simulink model "wlan_phy_tx_pmd"  (Simulink 7.8)
settings: Solver=VariableStepDiscrete  SolverMode=SingleTasking  StartTime=0.0  StopTime=inf  RelTol=1e-3
PostLoadFcn:
  | wlan_phy_tx_init
InitFcn:
  | wlan_phy_tx_init
StartFcn:
  | wlan_phy_tx_init
undefined symbols (not defined in the file): gcbh, ht_preamble_rom, MAX_CP_LEN, MAX_DATA_BITS_PER_SYM_PERIOD, MAX_NCBPS, MAX_NUM_BYTES, MAX_NUM_SC, MAX_NUM_SYMS, mcs_rom_11ag, mcs_rom_11n, Mod_Constellation_16QAM, Mod_Constellation_64QAM, Mod_Constellation_BPSK, Mod_Constellation_QPSK, Preamble_IQ, Preamble_IQ_scaled, tx_sim, wlan_tx_interleave_rom, xlBlockLoadCallback, xlGetNormalizedPeriod
libraries: xbsIndex_r4 x1358, xbsEDKLib_r4 x1
(part 7 of 10)

== system wlan_phy_tx_pmd/PSDU Syms Gen/Pkt Data/Packet Sections ==
  note: 11ag Bytes (L = SIGNAL.LENGTH):
      | 0:2        : SIGNAL       No FCS, Unscrambled
      | 3:4        : SERVICE      No FCS, Scrambled
      | 4:(L-5)    : MAC payload  FCS, Scrambled
      | (L-4):(L-1): FCS          Scrambled
      |            : PAD (zeros)  Unscrambled
      |            : TAIL (zeros) Scrambled
  note: 11n Bytes (L = HT-SIG.LENGTH):
      | 0:2        : SIGNAL       No FCS, Unscrambled
      | 3:8        : HT-SIG       No FCS, Unscrambled
      | 9:10       : SERVICE      No FCS, Scrambled
      | 10:(L-5)   : MAC payload  FCS, Scrambled
      | (L-4):(L-1): FCS          Scrambled
      |            : PAD (zeros)  Unscrambled
      |            : TAIL (zeros) Scrambled
  note: 6 bits past L are unscrambled zero (TAIL).
      | All further bits to fill symbol are scrambled
      | zeros (PAD).
  note: len(SIGNAL)
  note: len(L-SIG + HT-SIG)
  note: len(SERVICE)
  note: len(FCS)
  note: len(TAIL)
  Bit sel : Inport
  Byte Ind : Inport  Port=2
  AddSub1 : xbsIndex_r4/AddSub  mode=Addition  use_carryin=off  use_carryout=off  en=off  latency=1  precision=Full  arith_type=Unsigned  n_bits=ceil(log2(MAX_NUM_BYTES))  bin_pt=0  quantization=Truncate  overflow=Saturate  dbl_ovrd=off  use_behavioral_HDL=off  hw_selection=Fabric  pipelined=off  block_type=addsub
  AddSub2 : xbsIndex_r4/AddSub  mode=Subtraction  use_carryin=off  use_carryout=off  en=off  latency=1  precision=Full  arith_type=Unsigned  n_bits=ceil(log2(MAX_NUM_BYTES))  bin_pt=0  quantization=Truncate  overflow=Saturate  dbl_ovrd=off  use_behavioral_HDL=off  hw_selection=Fabric  pipelined=off  block_type=addsub
  AddSub3 : xbsIndex_r4/AddSub  mode=Addition  use_carryin=off  use_carryout=off  en=off  latency=1  precision=Full  arith_type=Unsigned  n_bits=ceil(log2(MAX_NUM_BYTES))  bin_pt=0  quantization=Truncate  overflow=Saturate  dbl_ovrd=off  use_behavioral_HDL=off  hw_selection=Fabric  pipelined=off  block_type=addsub
  Constant1 : xbsIndex_r4/Constant  const=3  gui_display_data_type=Fixed-point  arith_type=Unsigned  n_bits=3  bin_pt=0  preci_type=Single  exp_width=8  frac_width=24  explicit_period=off  period=1  equ=P=C  opselect=C  inp2=PCIN>>17  opr=+  inp1=P  carry=CIN  dbl_ovrd=off  block_type=constant
  Constant2 : xbsIndex_r4/Constant  const=9  gui_display_data_type=Fixed-point  arith_type=Unsigned  n_bits=4  bin_pt=0  preci_type=Single  exp_width=8  frac_width=24  explicit_period=off  period=1  equ=P=C  opselect=C  inp2=PCIN>>17  opr=+  inp1=P  carry=CIN  dbl_ovrd=off  block_type=constant
  Constant3 : xbsIndex_r4/Constant  const=4  gui_display_data_type=Fixed-point  arith_type=Unsigned  n_bits=3  bin_pt=0  preci_type=Single  exp_width=8  frac_width=24  explicit_period=off  period=1  equ=P=C  opselect=C  inp2=PCIN>>17  opr=+  inp1=P  carry=CIN  dbl_ovrd=off  block_type=constant
  Constant4 : xbsIndex_r4/Constant  const=6  gui_display_data_type=Fixed-point  arith_type=Unsigned  n_bits=3  bin_pt=0  preci_type=Single  exp_width=8  frac_width=24  explicit_period=off  period=1  equ=P=C  opselect=C  inp2=PCIN>>17  opr=+  inp1=P  carry=CIN  dbl_ovrd=off  block_type=constant
  Constant5 : xbsIndex_r4/Constant  const=2  gui_display_data_type=Fixed-point  arith_type=Unsigned  n_bits=3  bin_pt=0  preci_type=Single  exp_width=8  frac_width=24  explicit_period=off  period=1  equ=P=C  opselect=C  inp2=PCIN>>17  opr=+  inp1=P  carry=CIN  dbl_ovrd=off  block_type=constant
  Constant6 : xbsIndex_r4/Constant  const=9  gui_display_data_type=Fixed-point  arith_type=Unsigned  n_bits=4  bin_pt=0  preci_type=Single  exp_width=8  frac_width=24  explicit_period=off  period=1  equ=P=C  opselect=C  inp2=PCIN>>17  opr=+  inp1=P  carry=CIN  dbl_ovrd=off  block_type=constant
  Constant7 : xbsIndex_r4/Constant  const=3  gui_display_data_type=Fixed-point  arith_type=Unsigned  n_bits=4  bin_pt=0  preci_type=Single  exp_width=8  frac_width=24  explicit_period=off  period=1  equ=P=C  opselect=C  inp2=PCIN>>17  opr=+  inp1=P  carry=CIN  dbl_ovrd=off  block_type=constant
  DATA Sections : Scope  NumInputPorts=7
      settings: YMin=-5~-5~-5~-5~-5~-5~-5  YMax=5~5~5~5~5~5~5
  Display : Display
  Gateway Out{1..7} (7 alike) : xbsIndex_r4/Gateway Out  inherit_from_input=off  hdl_port=off  timing_constraint=None  locs_specified=off  LOCs={}  UseAsDAC=off  DACChannel='1'  block_type=gatewayout
  Inverter : xbsIndex_r4/Inverter  en=off  latency=0  dbl_ovrd=off  block_type=inv
  Inverter1 : xbsIndex_r4/Inverter  en=off  latency=0  dbl_ovrd=off  block_type=inv
  Logical1 : xbsIndex_r4/Logical  logical_function=OR  inputs=2  en=off  latency=0  precision=Full  arith_type=Unsigned  n_bits=16  bin_pt=0  align_bp=on  dbl_ovrd=off  block_type=logical
  Logical2 : xbsIndex_r4/Logical  logical_function=AND  inputs=2  en=off  latency=0  precision=Full  arith_type=Unsigned  n_bits=16  bin_pt=0  align_bp=on  dbl_ovrd=off  block_type=logical
  Logical3 : xbsIndex_r4/Logical  logical_function=AND  inputs=2  en=off  latency=0  precision=Full  arith_type=Unsigned  n_bits=16  bin_pt=0  align_bp=on  dbl_ovrd=off  block_type=logical
  Logical4 : xbsIndex_r4/Logical  logical_function=AND  inputs=2  en=off  latency=0  precision=Full  arith_type=Unsigned  n_bits=16  bin_pt=0  align_bp=on  dbl_ovrd=off  block_type=logical
  Logical5 : xbsIndex_r4/Logical  logical_function=AND  inputs=3  en=off  latency=0  precision=Full  arith_type=Unsigned  n_bits=16  bin_pt=0  align_bp=on  dbl_ovrd=off  block_type=logical
  Mux8 : xbsIndex_r4/Mux  inputs=2  en=off  latency=0  precision=Full  arith_type=Unsigned  n_bits=16  bin_pt=14  quantization=Truncate  overflow=Wrap  dbl_ovrd=off  block_type=mux
  Relational1 : xbsIndex_r4/Relational  mode=a>=b  en=off  latency=0  dbl_ovrd=off  block_type=relational
  Relational2 : xbsIndex_r4/Relational  mode=a<b  en=off  latency=0  dbl_ovrd=off  block_type=relational
  Relational3 : xbsIndex_r4/Relational  mode=a<b  en=off  latency=0  dbl_ovrd=off  block_type=relational
  Relational4 : xbsIndex_r4/Relational  mode=a>=b  en=off  latency=0  dbl_ovrd=off  block_type=relational
  Relational5 : xbsIndex_r4/Relational  mode=a=b  en=off  latency=0  dbl_ovrd=off  block_type=relational
  Relational6 : xbsIndex_r4/Relational  mode=a<b  en=off  latency=0  dbl_ovrd=off  block_type=relational
  Relational7 : xbsIndex_r4/Relational  mode=a>=b  en=off  latency=0  dbl_ovrd=off  block_type=relational
  Unscrambled : Outport
  Sel Zero : Outport  Port=2
  Sel FCS : Outport  Port=3
  Sel HTSIG : Outport  Port=4
  DATA Done : Outport  Port=5
  wires:
  Mux8/1 -> Relational2/2, AddSub3/1
  Relational2/1 -> Logical1/1  "SIG/HTSIG"
  Logical1/1 -> Unscrambled/1, Gateway Out2/1
  [OFDM_TX_DATA_LENGTH] -> AddSub1/2, Gateway Out4/1
  [Tx_PHY_Mode_11n] -> Mux8/1
  Constant1/1 -> Mux8/2
  Constant2/1 -> Mux8/3
  AddSub1/1 -> Relational5/2, Relational4/2, AddSub2/1
  Relational4/1 -> Inverter/1, Sel Zero/1, Gateway Out5/1  "PAD"
  Constant4/1 -> Relational6/2
  Logical4/1 -> Logical1/2  "TAIL"
  Relational6/1 -> Logical4/1, Inverter1/1
  Relational5/1 -> Logical4/2, Logical3/2
  Byte Ind/1 -> Relational2/1, Relational5/1, Relational4/1, Relational1/1, Relational3/1, Relational7/1, Gateway Out3/1
  Bit sel/1 -> Relational6/1, Gateway Out1/1
  Constant3/1 -> AddSub2/2
  AddSub2/1 -> Relational1/2
  Constant5/1 -> AddSub3/2
  AddSub3/1 -> AddSub1/1
  Inverter/1 -> Logical2/1
  Relational1/1 -> Logical2/2
  Logical2/1 -> Sel FCS/1, Gateway Out6/1
  Gateway Out1/1 -> DATA Sections/2  "Bit Sel"
  Gateway Out3/1 -> DATA Sections/1  "Byte Ind"
  Gateway Out2/1 -> DATA Sections/3  "Unscrambled"
  Gateway Out5/1 -> DATA Sections/4  "Sel Zero"
  Gateway Out4/1 -> Display/1
  Gateway Out6/1 -> DATA Sections/5  "Sel FCS"
  Gateway Out7/1 -> DATA Sections/6  "DATA Done"
  Logical3/1 -> DATA Done/1, Gateway Out7/1
  Inverter1/1 -> Logical3/1
  [Tx_PHY_Mode_11n] -> Logical5/1
  Constant6/1 -> Relational3/2
  Relational3/1 -> Logical5/2
  Relational7/1 -> Logical5/3
  Constant7/1 -> Relational7/2
  Logical5/1 -> Sel HTSIG/1

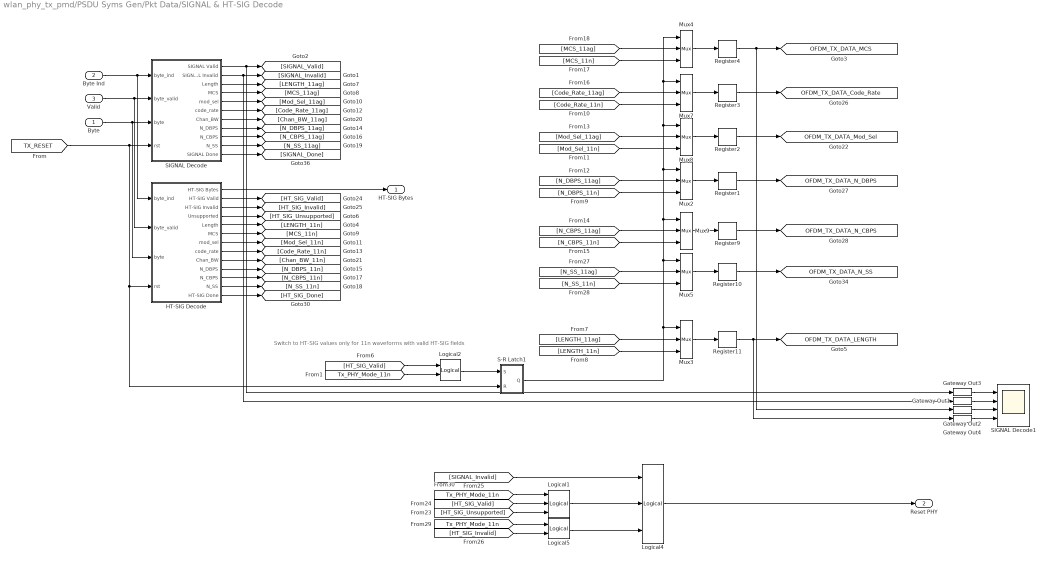
== system wlan_phy_tx_pmd/PSDU Syms Gen/Pkt Data/SIGNAL & HT-SIG Decode ==
  note: Switch to HT-SIG values only for
      | 11n waveforms with valid HT-SIG fields
  Byte : Inport
  Byte Ind : Inport  Port=2
  Valid : Inport  Port=3
  Gateway Out{1..4} (4 alike) : xbsIndex_r4/Gateway Out  inherit_from_input=off  hdl_port=off  timing_constraint=None  locs_specified=off  LOCs={}  UseAsDAC=off  DACChannel='1'  block_type=gatewayout
  HT-SIG Decode : Subsystem
  Logical1 : xbsIndex_r4/Logical  logical_function=AND  inputs=3  en=off  latency=0  precision=Full  arith_type=Unsigned  n_bits=16  bin_pt=0  align_bp=on  dbl_ovrd=off  block_type=logical
  Logical2 : xbsIndex_r4/Logical  logical_function=AND  inputs=2  en=off  latency=0  precision=Full  arith_type=Unsigned  n_bits=16  bin_pt=0  align_bp=on  dbl_ovrd=off  block_type=logical
  Logical4 : xbsIndex_r4/Logical  logical_function=OR  inputs=3  en=off  latency=0  precision=Full  arith_type=Unsigned  n_bits=16  bin_pt=0  align_bp=on  dbl_ovrd=off  block_type=logical
  Logical5 : xbsIndex_r4/Logical  logical_function=AND  inputs=2  en=off  latency=0  precision=Full  arith_type=Unsigned  n_bits=16  bin_pt=0  align_bp=on  dbl_ovrd=off  block_type=logical
  Mux{2..5,7..9} (7 alike) : xbsIndex_r4/Mux  inputs=2  en=off  latency=0  precision=Full  arith_type=Unsigned  n_bits=16  bin_pt=14  quantization=Truncate  overflow=Wrap  dbl_ovrd=off  block_type=mux
  Register{1..4,9..11} (7 alike) : xbsIndex_r4/Register  init=0  rst=off  en=off  dbl_ovrd=off  block_type=register
  S-R Latch1 : Subsystem
  SIGNAL Decode : Subsystem
  SIGNAL Decode1 : Scope  NumInputPorts=4
      settings: TimeRange=11440  YMin=-5~-5~-5~-5  YMax=5~5~5~5  SaveName=ScopeData2
  HT-SIG Bytes : Outport
  Reset PHY : Outport  Port=2
  tag scope: OFDM_TX_DATA_Code_Rate=global, OFDM_TX_DATA_LENGTH=global, OFDM_TX_DATA_MCS=global, OFDM_TX_DATA_Mod_Sel=global, OFDM_TX_DATA_N_CBPS=global, OFDM_TX_DATA_N_DBPS=global, OFDM_TX_DATA_N_SS=global
  wires:
  Byte Ind/1 -> SIGNAL Decode/1(byte_ind), HT-SIG Decode/1(byte_ind)
  Valid/1 -> SIGNAL Decode/2(byte_valid), HT-SIG Decode/2(byte_valid)
  Byte/1 -> SIGNAL Decode/3(byte), HT-SIG Decode/3(byte)
  [TX_RESET] -> SIGNAL Decode/4(rst), HT-SIG Decode/4(rst), S-R Latch1/2(R)
  SIGNAL Decode/3(Length) -> [LENGTH_11ag]
  SIGNAL Decode/4(MCS) -> [MCS_11ag]
  SIGNAL Decode/5(mod_sel) -> [Mod_Sel_11ag]
  SIGNAL Decode/1(SIGNAL Valid) -> [SIGNAL_Valid], Gateway Out3/1
  SIGNAL Decode/2(SIGNAL Invalid) -> [SIGNAL_Invalid], Gateway Out1/1
  SIGNAL Decode/6(code_rate) -> [Code_Rate_11ag]
  SIGNAL Decode/7(Chan_BW) -> [Chan_BW_11ag]
  SIGNAL Decode/8(N_DBPS) -> [N_DBPS_11ag]
  SIGNAL Decode/9(N_CBPS) -> [N_CBPS_11ag]
  SIGNAL Decode/10(N_SS) -> [N_SS_11ag]
  HT-SIG Decode/2(HT-SIG Valid) -> [HT_SIG_Valid]
  HT-SIG Decode/3(HT-SIG Invalid) -> [HT_SIG_Invalid]
  HT-SIG Decode/4(Unsupported) -> [HT_SIG_Unsupported]
  HT-SIG Decode/5(Length) -> [LENGTH_11n]
  HT-SIG Decode/6(MCS) -> [MCS_11n]
  HT-SIG Decode/7(mod_sel) -> [Mod_Sel_11n]
  HT-SIG Decode/8(code_rate) -> [Code_Rate_11n]
  HT-SIG Decode/9(Chan_BW) -> [Chan_BW_11n]
  HT-SIG Decode/10(N_DBPS) -> [N_DBPS_11n]
  HT-SIG Decode/11(N_CBPS) -> [N_CBPS_11n]
  HT-SIG Decode/12(N_SS) -> [N_SS_11n]
  Mux3/1 -> Register11/1
  [LENGTH_11ag] -> Mux3/2
  [LENGTH_11n] -> Mux3/3
  [Code_Rate_11ag] -> Mux7/2
  [Code_Rate_11n] -> Mux7/3
  Mux7/1 -> Register3/1
  [Mod_Sel_11ag] -> Mux8/2
  [Mod_Sel_11n] -> Mux8/3
  Mux8/1 -> Register2/1
  [N_DBPS_11ag] -> Mux2/2
  [N_DBPS_11n] -> Mux2/3
  Mux2/1 -> Register1/1
  [N_CBPS_11ag] -> Mux9/2
  [N_CBPS_11n] -> Mux9/3
  Mux9/1 -> Register9/1
  Logical2/1 -> S-R Latch1/1(S)
  S-R Latch1/1(Q) -> Mux3/1, Mux9/1, Mux2/1, Mux8/1, Mux7/1, Mux4/1, Mux5/1
  [MCS_11ag] -> Mux4/2
  [MCS_11n] -> Mux4/3
  Mux4/1 -> Register4/1
  HT-SIG Decode/13(HT-SIG Done) -> [HT_SIG_Done]
  [Tx_PHY_Mode_11n] -> Logical1/1
  [HT_SIG_Valid] -> Logical1/2
  [SIGNAL_Invalid] -> Logical4/1
  Logical5/1 -> Logical4/3
  Logical4/1 -> Reset PHY/1
  [N_SS_11ag] -> Mux5/2
  [N_SS_11n] -> Mux5/3
  Mux5/1 -> Register10/1
  [Tx_PHY_Mode_11n] -> Logical5/1
  [HT_SIG_Invalid] -> Logical5/2
  Logical1/1 -> Logical4/2
  [HT_SIG_Unsupported] -> Logical1/3
  SIGNAL Decode/11(SIGNAL Done) -> [SIGNAL_Done]
  Register1/1 -> [OFDM_TX_DATA_N_DBPS]
  Register2/1 -> [OFDM_TX_DATA_Mod_Sel]
  Register3/1 -> [OFDM_TX_DATA_Code_Rate]
  Register4/1 -> [OFDM_TX_DATA_MCS], Gateway Out2/1
  Register9/1 -> [OFDM_TX_DATA_N_CBPS]
  Register10/1 -> [OFDM_TX_DATA_N_SS]
  Register11/1 -> [OFDM_TX_DATA_LENGTH], Gateway Out4/1
  [Tx_PHY_Mode_11n] -> Logical2/2
  [HT_SIG_Valid] -> Logical2/1
  Gateway Out1/1 -> SIGNAL Decode1/2
  Gateway Out3/1 -> SIGNAL Decode1/1
  Gateway Out2/1 -> SIGNAL Decode1/3
  Gateway Out4/1 -> SIGNAL Decode1/4
  HT-SIG Decode/1(HT-SIG Bytes) -> HT-SIG Bytes/1

== system wlan_phy_tx_pmd/PSDU Syms Gen/Pkt Data/Scrambling ==
  note: Increment the LFSR once per scrambled bit. Unscrambled
      | bits do not update the LFSR state and are not XOR'd with
      | the LFSR output.
  Bit Valid : Inport
  Unscrambled : Inport  Port=2
  Bit : Inport  Port=3
  Convert2 : xbsIndex_r4/Convert  gui_display_data_type=Fixed-point  arith_type=Unsigned  n_bits=1  bin_pt=0  float_type=Single  exp_bits=8  fraction_bits=24  quantization=Truncate  overflow=Wrap  en=off  latency=0  dbl_ovrd=off  pipeline=off  block_type=convert
  Inverter1 : xbsIndex_r4/Inverter  en=off  latency=0  dbl_ovrd=off  block_type=inv
  Logical : xbsIndex_r4/Logical  logical_function=XOR  inputs=2  en=off  latency=0  precision=Full  arith_type=Unsigned  n_bits=16  bin_pt=0  align_bp=on  dbl_ovrd=off  block_type=logical
  Logical2 : xbsIndex_r4/Logical  logical_function=AND  inputs=2  en=off  latency=0  precision=Full  arith_type=Unsigned  n_bits=16  bin_pt=0  align_bp=on  dbl_ovrd=off  block_type=logical
  Logical3 : xbsIndex_r4/Logical  logical_function=AND  inputs=2  en=off  latency=0  precision=Full  arith_type=Unsigned  n_bits=16  bin_pt=0  align_bp=on  dbl_ovrd=off  block_type=logical
  Scrambling LFSR : Subsystem
  Tx Bit : Outport
  wires:
  Inverter1/1 -> Logical2/2, Convert2/1
  Logical2/1 -> Scrambling LFSR/1(en)
  Scrambling LFSR/1(Q) -> Logical3/1
  Logical3/1 -> Logical/1
  Logical/1 -> Tx Bit/1
  Bit Valid/1 -> Logical2/1
  Unscrambled/1 -> Inverter1/1
  Bit/1 -> Logical/2
  Convert2/1 -> Logical3/2

== system wlan_phy_tx_pmd/PSDU Syms Gen/Pkt Data/negedge ==
  D : Inport
  Delay : xbsIndex_r4/Delay  rst=off  infoeditControl=Selection of Reset will increase slice count due to use of real FFs and instead of SRLs  en=off  latency=1  dbl_ovrd=off  reg_retiming=off  block_type=delay
      settings: infoedit=Hardware notes: A delay line is a chain, each link of which is an SRL16 followed by a flip-flop. If register retiming is enabled, the delay line is a chain of flip-flops.  xl_area=[1 1 0 0 0 0 0]  block_version=VER_STRING_GOES_HERE
  Inverter : xbsIndex_r4/Inverter  en=off  latency=0  dbl_ovrd=off  block_type=inv
      settings: xl_area=[0 0 0 0 0 0 0]  block_version=VER_STRING_GOES_HERE
  Logical1 : xbsIndex_r4/Logical  logical_function=AND  inputs=2  en=off  latency=0  precision=Full  arith_type=Unsigned  n_bits=8  bin_pt=2  align_bp=on  dbl_ovrd=off  block_type=logical
      settings: xl_area=[1 0 0 1 0 0 0]  block_version=VER_STRING_GOES_HERE
  Q : Outport
  wires:
  Logical1/1 -> Q/1
  D/1 -> Delay/1, Inverter/1
  Inverter/1 -> Logical1/1
  Delay/1 -> Logical1/2

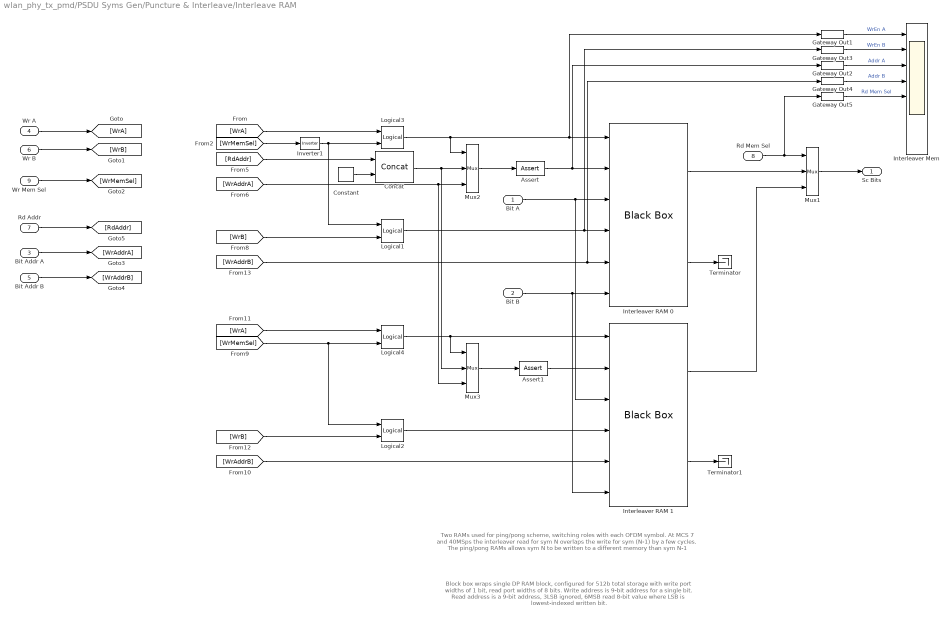
== system wlan_phy_tx_pmd/PSDU Syms Gen/Puncture & Interleave/Interleave RAM ==
  note: Block box wraps single DP RAM block, configured for 512b total storage with write port widths of 1 bit,
      | read port widths of 8 bits.
      |
      | Write address is 9-bit address for a single bit.
      |
      | Read address is a 9-bit address, 3LSB ignored, 6MSB read 8-bit value where LSB is lowest-indexed written bit.
  note: Two RAMs used for ping/pong scheme, switching roles with each OFDM symbol. At MCS 7 and 40MSps
      | the interleaver read for sym N overlaps the write for sym (N-1) by a few cycles. The ping/pong RAMs allows
      | sym N to be written to a different memory than sym N-1
  Bit A : Inport
  Bit B : Inport  Port=2
  Bit Addr A : Inport  Port=3
  Wr A : Inport  Port=4
  Bit Addr B : Inport  Port=5
  Wr B : Inport  Port=6
  Rd Addr : Inport  Port=7
  Rd Mem Sel : Inport  Port=8
  Wr Mem Sel : Inport  Port=9
  Assert : xbsIndex_r4/Assert  assert_type=on  type_source=Explicitly  gui_display_data_type=Fixed-point  arith_type=Unsigned  n_bits=9  bin_pt=0  preci_type=Single  exp_width=8  frac_width=24  assert_rate=on  rate_source=Explicitly  period=1  output_port=on  block_type=assert
  Assert1 : xbsIndex_r4/Assert  assert_type=on  type_source=Explicitly  gui_display_data_type=Fixed-point  arith_type=Unsigned  n_bits=9  bin_pt=0  preci_type=Single  exp_width=8  frac_width=24  assert_rate=on  rate_source=Explicitly  period=1  output_port=on  block_type=assert
  Concat : xbsIndex_r4/Concat  num_inputs=2  dbl_ovrd=off  block_type=concat
  Constant : xbsIndex_r4/Constant  const=0  gui_display_data_type=Fixed-point  arith_type=Unsigned  n_bits=3  bin_pt=0  preci_type=Single  exp_width=8  frac_width=24  explicit_period=off  period=1  equ=P=C  opselect=C  inp2=PCIN>>17  opr=+  inp1=P  carry=CIN  dbl_ovrd=off  block_type=constant
  Gateway Out{1..5} (5 alike) : xbsIndex_r4/Gateway Out  inherit_from_input=off  hdl_port=off  timing_constraint=None  locs_specified=off  LOCs={}  UseAsDAC=off  DACChannel='1'  block_type=gatewayout
  Interleaver Mem : Scope  NumInputPorts=8
      settings: TimeRange=25000  YMin=0~0~0~0~0~-1~-1~-1  YMax=1~1~500~500~1~1~1~1  SaveName=ScopeData9
  Interleaver RAM 0 : xbsIndex_r4/Black Box  init_code=interleaver_ram  sim_method=ISE Simulator  verbose=off  block_type=blackbox2
  Interleaver RAM 1 : xbsIndex_r4/Black Box  init_code=interleaver_ram  sim_method=ISE Simulator  verbose=off  block_type=blackbox2
  Inverter1 : xbsIndex_r4/Inverter  en=off  latency=0  dbl_ovrd=off  block_type=inv
  Logical{1..4} (4 alike) : xbsIndex_r4/Logical  logical_function=AND  inputs=2  en=off  latency=0  precision=Full  arith_type=Unsigned  n_bits=16  bin_pt=0  align_bp=on  dbl_ovrd=off  block_type=logical
  Mux1 : xbsIndex_r4/Mux  inputs=2  en=off  latency=0  precision=Full  arith_type=Unsigned  n_bits=16  bin_pt=14  quantization=Truncate  overflow=Wrap  dbl_ovrd=off  block_type=mux
  Mux2 : xbsIndex_r4/Mux  inputs=2  en=off  latency=0  precision=Full  arith_type=Unsigned  n_bits=16  bin_pt=14  quantization=Truncate  overflow=Wrap  dbl_ovrd=off  block_type=mux
  Mux3 : xbsIndex_r4/Mux  inputs=2  en=off  latency=0  precision=Full  arith_type=Unsigned  n_bits=16  bin_pt=14  quantization=Truncate  overflow=Wrap  dbl_ovrd=off  block_type=mux
  Terminator : Terminator
  Terminator1 : Terminator
  Sc Bits : Outport
  wires:
  Logical3/1 -> Mux2/1, Interleaver RAM 0/1, Gateway Out1/1
  Interleaver RAM 0/1 -> Mux1/2
  Interleaver RAM 0/2 -> Terminator/1
  [WrAddrA] -> Mux2/3, Mux3/3
  Mux2/1 -> Assert/1
  [RdAddr] -> Concat/1
  Constant/1 -> Concat/2
  Concat/1 -> Mux2/2, Mux3/2
  Gateway Out1/1 -> Interleaver Mem/1  "WrEn A"
  Gateway Out3/1 -> Interleaver Mem/2  "WrEn B"
  Gateway Out2/1 -> Interleaver Mem/3  "Addr A"
  Gateway Out4/1 -> Interleaver Mem/4  "Addr B"
  Interleaver RAM 1/2 -> Terminator1/1
  Mux1/1 -> Sc Bits/1
  Interleaver RAM 1/1 -> Mux1/3
  Rd Mem Sel/1 -> Mux1/1, Gateway Out5/1
  Gateway Out5/1 -> Interleaver Mem/5  "Rd Mem Sel"
  Wr A/1 -> [WrA]
  Wr B/1 -> [WrB]
  Wr Mem Sel/1 -> [WrMemSel]
  Bit Addr B/1 -> [WrAddrB]
  Rd Addr/1 -> [RdAddr]
  Bit Addr A/1 -> [WrAddrA]
  [WrA] -> Logical3/1
  [WrMemSel] -> Inverter1/1
  Inverter1/1 -> Logical3/2, Logical1/1
  Logical4/1 -> Interleaver RAM 1/1, Mux3/1
  [WrA] -> Logical4/1
  [WrMemSel] -> Logical4/2, Logical2/1
  Mux3/1 -> Assert1/1
  Assert/1 -> Interleaver RAM 0/2, Gateway Out2/1
  Assert1/1 -> Interleaver RAM 1/2
  [WrAddrB] -> Interleaver RAM 1/5
  Bit A/1 -> Interleaver RAM 0/3, Interleaver RAM 1/3
  Bit B/1 -> Interleaver RAM 0/6, Interleaver RAM 1/6
  Logical1/1 -> Interleaver RAM 0/4, Gateway Out3/1
  Logical2/1 -> Interleaver RAM 1/4
  [WrAddrB] -> Interleaver RAM 0/5, Gateway Out4/1
  [WrB] -> Logical1/2
  [WrB] -> Logical2/2

== system wlan_phy_tx_pmd/PSDU Syms Gen/Puncture & Interleave/Interleaver Ctrl & Puncturing ==
  note: The code puncturing is implemented as part of the interleaver. The
      | interleaver RAM can record 2 coded bits per cycle (the A and B outputs
      | of the convolutional encoder). A coded bit is punctured by not being
      | written to the interleaver RAM.
      |
      | This interleaver design operates at the effective rate of 1 uncoded data bit
      | per cycle, allowing the overall architecture to achieve a data rate equal
      | to the master clock frequency. This is achieved by writing 2 coded bits
      | per cycle to the interleave RAM (2 coded bits = 1 data bit). It would be
      | simpler to serialize the coded bits, but this would cut the max data rate
      | in half, which would complicate implementation of HT40 and N_SS=2 modes
      | in the future.
      |
      | The interleaver RAM outputs coded bits in groups. The number of valid
      | bits in each group equals the number of coded bits in a subcarrier for
      | the current symbol's MCS. This architecture (write 2 bits per cycle, read all
      | bits for a subcarrier in 1 cycle) minimizes latency through the interleaver.
  Bits tvalid : Inport
  Base Rate : Inport  Port=2
  Bit Index Calc : Subsystem
  Constant2 : xbsIndex_r4/Constant  const=0  gui_display_data_type=Fixed-point  arith_type=Unsigned  n_bits=2  bin_pt=0  preci_type=Single  exp_width=8  frac_width=24  explicit_period=off  period=1  equ=P=C  opselect=C  inp2=PCIN>>17  opr=+  inp1=P  carry=CIN  dbl_ovrd=off  block_type=constant
  Delay1 : xbsIndex_r4/Delay  rst=off  infoeditControl=Selection of Reset will increase slice count due to use of real FFs and instead of SRLs  en=off  latency=1  dbl_ovrd=off  reg_retiming=off  block_type=delay
  Delay2 : xbsIndex_r4/Delay  rst=off  infoeditControl=Selection of Reset will increase slice count due to use of real FFs and instead of SRLs  en=off  latency=1  dbl_ovrd=off  reg_retiming=off  block_type=delay
  Gateway Out{1..8} (8 alike) : xbsIndex_r4/Gateway Out  inherit_from_input=off  hdl_port=off  timing_constraint=None  locs_specified=off  LOCs={}  UseAsDAC=off  DACChannel='1'  block_type=gatewayout
  Interleave Mapping : Subsystem
  Interleaver Control : Scope  NumInputPorts=8
      settings: TimeRange=5000  YMin=0~0~0~0~0~0~0~0  YMax=1~1~1~1~400~400~500~500  SaveName=ScopeData38
  Logical2 : xbsIndex_r4/Logical  logical_function=OR  inputs=2  en=off  latency=0  precision=Full  arith_type=Unsigned  n_bits=16  bin_pt=0  align_bp=on  dbl_ovrd=off  block_type=logical
  Mux2 : xbsIndex_r4/Mux  inputs=2  en=off  latency=0  precision=Full  arith_type=Unsigned  n_bits=16  bin_pt=14  quantization=Truncate  overflow=Wrap  dbl_ovrd=off  block_type=mux
  Puncturing : Subsystem
  negedge : Subsystem
  Addr A : Outport
  Wr A : Outport  Port=2
  Addr B : Outport  Port=3
  Wr B : Outport  Port=4
  wires:
  Puncturing/1(Index Inc) -> Bit Index Calc/1(Inc)
  Gateway Out1/1 -> Interleaver Control/1  "Rate"
  Gateway Out4/1 -> Interleaver Control/4  "En"
  Gateway Out5/1 -> Interleaver Control/5  "Ind A"
  Mux2/1 -> Puncturing/1(Code Rate), Gateway Out1/1
  Logical2/1 -> Bit Index Calc/2(Rst), Gateway Out8/1, Puncturing/2(Reset)
  Bits tvalid/1 -> negedge/1(D), Bit Index Calc/3(En), Gateway Out4/1, Puncturing/3(En)
  Bit Index Calc/1(Ind A) -> Gateway Out5/1, Interleave Mapping/2(Ind A)  "Ind A"
  Bit Index Calc/2(Ind B) -> Gateway Out6/1, Interleave Mapping/3(Ind B)  "Ind B"
  Gateway Out6/1 -> Interleaver Control/6  "Ind B"
  Puncturing/2(Wr A) -> Delay1/1
  Puncturing/3(Wr B) -> Delay2/1
  Base Rate/1 -> Mux2/1, Interleave Mapping/1(Base Rate Sym), Gateway Out3/1
  Constant2/1 -> Mux2/3
  [OFDM_TX_DATA_Code_Rate] -> Mux2/2
  Gateway Out3/1 -> Interleaver Control/2  "Base Rate"
  Delay1/1 -> Wr A/1
  Delay2/1 -> Wr B/1
  Interleave Mapping/1(Addr A) -> Addr A/1, Gateway Out2/1
  Interleave Mapping/2(Addr B) -> Addr B/1, Gateway Out7/1
  negedge/1(Q) -> Logical2/2
  [TX_RESET] -> Logical2/1
  Gateway Out2/1 -> Interleaver Control/7  "Addr A"
  Gateway Out7/1 -> Interleaver Control/8  "Addr B"
  Gateway Out8/1 -> Interleaver Control/3  "Reset"

== system wlan_phy_tx_pmd/PSDU Syms Gen/Puncture & Interleave/Mem Sel ==
  note: Simple circuit to toggle between 0 and 1 each time the En signal asserts.
  En : Inport
  Inverter : xbsIndex_r4/Inverter  en=off  latency=0  dbl_ovrd=off  block_type=inv
  Logical : xbsIndex_r4/Logical  logical_function=AND  inputs=2  en=off  latency=0  precision=Full  arith_type=Unsigned  n_bits=16  bin_pt=0  align_bp=on  dbl_ovrd=off  block_type=logical
  Logical1 : xbsIndex_r4/Logical  logical_function=AND  inputs=2  en=off  latency=0  precision=Full  arith_type=Unsigned  n_bits=16  bin_pt=0  align_bp=on  dbl_ovrd=off  block_type=logical
  Logical2 : xbsIndex_r4/Logical  logical_function=OR  inputs=2  en=off  latency=0  precision=Full  arith_type=Unsigned  n_bits=16  bin_pt=0  align_bp=on  dbl_ovrd=off  block_type=logical
  S-R Latch1 : Subsystem
  Rd : Outport
  Wr : Outport  Port=2
  wires:
  S-R Latch1/1(Q) -> Inverter/1, Rd/1, Logical1/2
  Logical2/1 -> S-R Latch1/2(R)
  Logical/1 -> S-R Latch1/1(S)
  Inverter/1 -> Wr/1, Logical/1
  En/1 -> Logical/2, Logical1/1
  Logical1/1 -> Logical2/1
  [TX_RESET] -> Logical2/2

== system wlan_phy_tx_pmd/Preamble & Outputs/DAC Outputs/Ant Enables ==
  Logical{1,3,5,7} (4 alike) : xbsIndex_r4/Logical  logical_function=AND  inputs=2  en=off  latency=0  precision=Full  arith_type=Unsigned  n_bits=16  bin_pt=0  align_bp=on  dbl_ovrd=off  block_type=logical
  Logical{2,4,6,8} (4 alike) : xbsIndex_r4/Logical  logical_function=OR  inputs=2  en=off  latency=0  precision=Full  arith_type=Unsigned  n_bits=16  bin_pt=0  align_bp=on  dbl_ovrd=off  block_type=logical
  b0 : xbsIndex_r4/Slice  nbits=1  boolean_output=on  mode=Lower Bit Location + Width  bit1=0  base1=MSB of Input  bit0=0  base0=LSB of Input  dbl_ovrd=off  block_type=slice
  b1 : xbsIndex_r4/Slice  nbits=1  boolean_output=on  mode=Lower Bit Location + Width  bit1=0  base1=MSB of Input  bit0=1  base0=LSB of Input  dbl_ovrd=off  block_type=slice
  b2 : xbsIndex_r4/Slice  nbits=1  boolean_output=on  mode=Lower Bit Location + Width  bit1=0  base1=MSB of Input  bit0=2  base0=LSB of Input  dbl_ovrd=off  block_type=slice
  b3 : xbsIndex_r4/Slice  nbits=1  boolean_output=on  mode=Lower Bit Location + Width  bit1=0  base1=MSB of Input  bit0=3  base0=LSB of Input  dbl_ovrd=off  block_type=slice
  A En : Outport
  B En : Outport  Port=2
  C En : Outport  Port=3
  D En : Outport  Port=4
  wires:
  [regTx_AntA_Tx_En] -> Logical2/1
  Logical2/1 -> A En/1
  [MAC_Tx_Ant_Mask] -> b0/1, b1/1, b2/1, b3/1
  Logical1/1 -> Logical2/2
  [regTx_Use_MAC_Ant_Masks] -> Logical1/2, Logical3/2, Logical5/2, Logical7/2
  b0/1 -> Logical1/1
  Logical3/1 -> Logical4/2
  [regTx_AntB_Tx_En] -> Logical4/1
  b1/1 -> Logical3/1
  Logical5/1 -> Logical6/2
  [regTx_AntC_Tx_En] -> Logical6/1
  b2/1 -> Logical5/1
  Logical7/1 -> Logical8/2
  [regTx_AntD_Tx_En] -> Logical8/1
  Logical4/1 -> B En/1
  Logical6/1 -> C En/1
  b3/1 -> Logical7/1
  Logical8/1 -> D En/1

== system wlan_phy_tx_pmd/Preamble & Outputs/End of Tx Ctrl/Posedge ==
  D : Inport
  Delay : xbsIndex_r4/Delay  rst=off  infoeditControl=Selection of Reset will increase slice count due to use of real FFs and instead of SRLs  en=off  latency=1  dbl_ovrd=off  reg_retiming=off  block_type=delay
      settings: infoedit=Hardware notes: A delay line is a chain, each link of which is an SRL16 followed by a flip-flop. If register retiming is enabled, the delay line is a chain of flip-flops.  xl_area=[1 1 0 0 0 0 0]  block_version=VER_STRING_GOES_HERE
  Inverter : xbsIndex_r4/Inverter  en=off  latency=0  dbl_ovrd=off  block_type=inv
      settings: xl_area=[0 0 0 0 0 0 0]  block_version=VER_STRING_GOES_HERE
  Logical1 : xbsIndex_r4/Logical  logical_function=AND  inputs=2  en=off  latency=0  precision=Full  arith_type=Unsigned  n_bits=8  bin_pt=2  align_bp=on  dbl_ovrd=off  block_type=logical
      settings: xl_area=[1 0 0 1 0 0 0]  block_version=VER_STRING_GOES_HERE
  Q : Outport
  wires:
  D/1 -> Logical1/2, Delay/1
  Logical1/1 -> Q/1
  Inverter/1 -> Logical1/1
  Delay/1 -> Inverter/1

== system wlan_phy_tx_pmd/Preamble & Outputs/End of Tx Ctrl/Posedge1 ==
  D : Inport
  Delay : xbsIndex_r4/Delay  rst=off  infoeditControl=Selection of Reset will increase slice count due to use of real FFs and instead of SRLs  en=off  latency=1  dbl_ovrd=off  reg_retiming=off  block_type=delay
      settings: infoedit=Hardware notes: A delay line is a chain, each link of which is an SRL16 followed by a flip-flop. If register retiming is enabled, the delay line is a chain of flip-flops.  xl_area=[1 1 0 0 0 0 0]  block_version=VER_STRING_GOES_HERE
  Inverter : xbsIndex_r4/Inverter  en=off  latency=0  dbl_ovrd=off  block_type=inv
      settings: xl_area=[0 0 0 0 0 0 0]  block_version=VER_STRING_GOES_HERE
  Logical1 : xbsIndex_r4/Logical  logical_function=AND  inputs=2  en=off  latency=0  precision=Full  arith_type=Unsigned  n_bits=8  bin_pt=2  align_bp=on  dbl_ovrd=off  block_type=logical
      settings: xl_area=[1 0 0 1 0 0 0]  block_version=VER_STRING_GOES_HERE
  Q : Outport
  wires:
  Delay/1 -> Inverter/1
  Inverter/1 -> Logical1/1
  Logical1/1 -> Q/1
  D/1 -> Delay/1, Logical1/2

== system wlan_phy_tx_pmd/Preamble & Outputs/End of Tx Ctrl/S-R Latch ==
  S : Inport
  R : Inport  Port=2
  Constant1 : xbsIndex_r4/Constant  const=1  gui_display_data_type=Fixed-point  arith_type=Boolean  n_bits=1  bin_pt=0  preci_type=Single  exp_width=8  frac_width=24  explicit_period=off  period=1  equ=P=C  opselect=C  inp2=PCIN>>17  opr=+  inp1=P  carry=CIN  dbl_ovrd=off  block_type=constant
      settings: block_version=VER_STRING_GOES_HERE
  Convert1 : xbsIndex_r4/Convert  gui_display_data_type=Boolean  arith_type=Boolean  n_bits=1  bin_pt=0  float_type=Single  exp_bits=8  fraction_bits=24  quantization=Truncate  overflow=Wrap  en=off  latency=0  dbl_ovrd=off  pipeline=off  block_type=convert
  Convert2 : xbsIndex_r4/Convert  gui_display_data_type=Boolean  arith_type=Boolean  n_bits=1  bin_pt=0  float_type=Single  exp_bits=8  fraction_bits=24  quantization=Truncate  overflow=Wrap  en=off  latency=0  dbl_ovrd=off  pipeline=off  block_type=convert
  Register2 : xbsIndex_r4/Register  init=0  rst=on  en=on  dbl_ovrd=off  block_type=register
      settings: xl_area=[1 1 0 0 0 0 0]  block_version=VER_STRING_GOES_HERE
  Q : Outport
  wires:
  Convert2/1 -> Register2/3
  Convert1/1 -> Register2/2
  Constant1/1 -> Register2/1
  R/1 -> Convert1/1
  Register2/1 -> Q/1
  S/1 -> Convert2/1

== system wlan_phy_tx_pmd/Preamble & Outputs/FIFO/I/Q Concat ==
  I : Inport
  Q : Inport  Port=2
  Concat : xbsIndex_r4/Concat  num_inputs=2  dbl_ovrd=off  block_type=concat
  Convert : xbsIndex_r4/Convert  gui_display_data_type=Fixed-point  arith_type="Signed  (2's comp)"  n_bits=16  bin_pt=15  float_type=Single  exp_bits=8  fraction_bits=24  quantization=Truncate  overflow=Saturate  en=off  latency=0  dbl_ovrd=off  pipeline=off  block_type=convert
  Convert1 : xbsIndex_r4/Convert  gui_display_data_type=Fixed-point  arith_type="Signed  (2's comp)"  n_bits=16  bin_pt=15  float_type=Single  exp_bits=8  fraction_bits=24  quantization=Truncate  overflow=Saturate  en=off  latency=0  dbl_ovrd=off  pipeline=off  block_type=convert
  FFT Clip : Scope  NumInputPorts=4
      settings: TimeRange=30000  YMin=0~0~0~-0.1  YMax=300~300~1~1.1  SaveName=ScopeData11
  Gateway Out{1..3,14} (4 alike) : xbsIndex_r4/Gateway Out  inherit_from_input=off  hdl_port=off  timing_constraint=None  locs_specified=off  LOCs={}  UseAsDAC=off  DACChannel='1'  block_type=gatewayout
  Reinterpret : xbsIndex_r4/Reinterpret  force_arith_type=on  arith_type=Unsigned  force_bin_pt=on  bin_pt=0  block_type=reinterpret
  Reinterpret1 : xbsIndex_r4/Reinterpret  force_arith_type=on  arith_type=Unsigned  force_bin_pt=on  bin_pt=0  block_type=reinterpret
  IQ : Outport
  wires:
  Q/1 -> Convert1/1, Gateway Out1/1
  Concat/1 -> IQ/1
  I/1 -> Convert/1, Gateway Out14/1
  Reinterpret1/1 -> Concat/2
  Reinterpret/1 -> Concat/1
  Convert/1 -> Reinterpret/1, Gateway Out3/1
  Convert1/1 -> Reinterpret1/1, Gateway Out2/1
  Gateway Out14/1 -> FFT Clip/1
  Gateway Out1/1 -> FFT Clip/2
  Gateway Out3/1 -> FFT Clip/3
  Gateway Out2/1 -> FFT Clip/4

== system wlan_phy_tx_pmd/Preamble & Outputs/FIFO/I/Q Slice ==
  IQ : Inport
  Reinterpret2 : xbsIndex_r4/Reinterpret  force_arith_type=on  arith_type="Signed  (2's comp)"  force_bin_pt=on  bin_pt=15  block_type=reinterpret
  Reinterpret3 : xbsIndex_r4/Reinterpret  force_arith_type=on  arith_type="Signed  (2's comp)"  force_bin_pt=on  bin_pt=15  block_type=reinterpret
  Slice : xbsIndex_r4/Slice  nbits=16  boolean_output=off  mode=Upper Bit Location + Width  bit1=0  base1=MSB of Input  bit0=0  base0=LSB of Input  dbl_ovrd=off  block_type=slice
  Slice1 : xbsIndex_r4/Slice  nbits=16  boolean_output=off  mode=Lower Bit Location + Width  bit1=0  base1=MSB of Input  bit0=0  base0=LSB of Input  dbl_ovrd=off  block_type=slice
  I : Outport
  Q : Outport  Port=2
  wires:
  Slice/1 -> Reinterpret2/1
  Slice1/1 -> Reinterpret3/1
  IQ/1 -> Slice1/1, Slice/1
  Reinterpret2/1 -> I/1
  Reinterpret3/1 -> Q/1

== system wlan_phy_tx_pmd/Start Ctrl/Add MAC Extension/S-R Latch1 ==
  S : Inport
  R : Inport  Port=2
  Constant1 : xbsIndex_r4/Constant  const=1  gui_display_data_type=Fixed-point  arith_type=Boolean  n_bits=1  bin_pt=0  preci_type=Single  exp_width=8  frac_width=24  explicit_period=off  period=1  equ=P=C  opselect=C  inp2=PCIN>>17  opr=+  inp1=P  carry=CIN  dbl_ovrd=off  block_type=constant
      settings: block_version=VER_STRING_GOES_HERE
  Convert1 : xbsIndex_r4/Convert  gui_display_data_type=Boolean  arith_type=Boolean  n_bits=1  bin_pt=0  float_type=Single  exp_bits=8  fraction_bits=24  quantization=Truncate  overflow=Wrap  en=off  latency=0  dbl_ovrd=off  pipeline=off  block_type=convert
  Convert2 : xbsIndex_r4/Convert  gui_display_data_type=Boolean  arith_type=Boolean  n_bits=1  bin_pt=0  float_type=Single  exp_bits=8  fraction_bits=24  quantization=Truncate  overflow=Wrap  en=off  latency=0  dbl_ovrd=off  pipeline=off  block_type=convert
  Register2 : xbsIndex_r4/Register  init=0  rst=on  en=on  dbl_ovrd=off  block_type=register
      settings: xl_area=[1 1 0 0 0 0 0]  block_version=VER_STRING_GOES_HERE
  Q : Outport
  wires:
  Constant1/1 -> Register2/1
  R/1 -> Convert1/1
  Register2/1 -> Q/1
  S/1 -> Convert2/1
  Convert1/1 -> Register2/2
  Convert2/1 -> Register2/3

== system wlan_phy_tx_pmd/Start Ctrl/Add MAC Extension/S-R Latch2 ==
  S : Inport
  R : Inport  Port=2
  Constant1 : xbsIndex_r4/Constant  const=1  gui_display_data_type=Fixed-point  arith_type=Boolean  n_bits=1  bin_pt=0  preci_type=Single  exp_width=8  frac_width=24  explicit_period=off  period=1  equ=P=C  opselect=C  inp2=PCIN>>17  opr=+  inp1=P  carry=CIN  dbl_ovrd=off  block_type=constant
      settings: block_version=VER_STRING_GOES_HERE
  Convert1 : xbsIndex_r4/Convert  gui_display_data_type=Boolean  arith_type=Boolean  n_bits=1  bin_pt=0  float_type=Single  exp_bits=8  fraction_bits=24  quantization=Truncate  overflow=Wrap  en=off  latency=0  dbl_ovrd=off  pipeline=off  block_type=convert
  Convert2 : xbsIndex_r4/Convert  gui_display_data_type=Boolean  arith_type=Boolean  n_bits=1  bin_pt=0  float_type=Single  exp_bits=8  fraction_bits=24  quantization=Truncate  overflow=Wrap  en=off  latency=0  dbl_ovrd=off  pipeline=off  block_type=convert
  Register2 : xbsIndex_r4/Register  init=0  rst=on  en=on  dbl_ovrd=off  block_type=register
      settings: xl_area=[1 1 0 0 0 0 0]  block_version=VER_STRING_GOES_HERE
  Q : Outport
  wires:
  Convert2/1 -> Register2/3
  Convert1/1 -> Register2/2
  S/1 -> Convert2/1
  Register2/1 -> Q/1
  R/1 -> Convert1/1
  Constant1/1 -> Register2/1

== system wlan_phy_tx_pmd/Start Ctrl/Add TXEN Extension/Posedge1 ==
  D : Inport
  Delay : xbsIndex_r4/Delay  rst=off  infoeditControl=Selection of Reset will increase slice count due to use of real FFs and instead of SRLs  en=off  latency=1  dbl_ovrd=off  reg_retiming=off  block_type=delay
      settings: infoedit=Hardware notes: A delay line is a chain, each link of which is an SRL16 followed by a flip-flop. If register retiming is enabled, the delay line is a chain of flip-flops.  xl_area=[1 1 0 0 0 0 0]  block_version=VER_STRING_GOES_HERE
  Inverter : xbsIndex_r4/Inverter  en=off  latency=0  dbl_ovrd=off  block_type=inv
      settings: xl_area=[0 0 0 0 0 0 0]  block_version=VER_STRING_GOES_HERE
  Logical1 : xbsIndex_r4/Logical  logical_function=AND  inputs=2  en=off  latency=0  precision=Full  arith_type=Unsigned  n_bits=8  bin_pt=2  align_bp=on  dbl_ovrd=off  block_type=logical
      settings: xl_area=[1 0 0 1 0 0 0]  block_version=VER_STRING_GOES_HERE
  Q : Outport
  wires:
  Delay/1 -> Inverter/1
  Inverter/1 -> Logical1/1
  Logical1/1 -> Q/1
  D/1 -> Delay/1, Logical1/2

== system wlan_phy_tx_pmd/Start Ctrl/Add TXEN Extension/Posedge2 ==
  D : Inport
  Delay : xbsIndex_r4/Delay  rst=off  infoeditControl=Selection of Reset will increase slice count due to use of real FFs and instead of SRLs  en=off  latency=1  dbl_ovrd=off  reg_retiming=off  block_type=delay
      settings: infoedit=Hardware notes: A delay line is a chain, each link of which is an SRL16 followed by a flip-flop. If register retiming is enabled, the delay line is a chain of flip-flops.  xl_area=[1 1 0 0 0 0 0]  block_version=VER_STRING_GOES_HERE
  Inverter : xbsIndex_r4/Inverter  en=off  latency=0  dbl_ovrd=off  block_type=inv
      settings: xl_area=[0 0 0 0 0 0 0]  block_version=VER_STRING_GOES_HERE
  Logical1 : xbsIndex_r4/Logical  logical_function=AND  inputs=2  en=off  latency=0  precision=Full  arith_type=Unsigned  n_bits=8  bin_pt=2  align_bp=on  dbl_ovrd=off  block_type=logical
      settings: xl_area=[1 0 0 1 0 0 0]  block_version=VER_STRING_GOES_HERE
  Q : Outport
  wires:
  D/1 -> Logical1/2, Delay/1
  Logical1/1 -> Q/1
  Inverter/1 -> Logical1/1
  Delay/1 -> Inverter/1

== system wlan_phy_tx_pmd/Start Ctrl/Add TXEN Extension/Posedge3 ==
  D : Inport
  Delay : xbsIndex_r4/Delay  rst=off  infoeditControl=Selection of Reset will increase slice count due to use of real FFs and instead of SRLs  en=off  latency=1  dbl_ovrd=off  reg_retiming=off  block_type=delay
      settings: infoedit=Hardware notes: A delay line is a chain, each link of which is an SRL16 followed by a flip-flop. If register retiming is enabled, the delay line is a chain of flip-flops.  xl_area=[1 1 0 0 0 0 0]  block_version=VER_STRING_GOES_HERE
  Inverter : xbsIndex_r4/Inverter  en=off  latency=0  dbl_ovrd=off  block_type=inv
      settings: xl_area=[0 0 0 0 0 0 0]  block_version=VER_STRING_GOES_HERE
  Logical1 : xbsIndex_r4/Logical  logical_function=AND  inputs=2  en=off  latency=0  precision=Full  arith_type=Unsigned  n_bits=8  bin_pt=2  align_bp=on  dbl_ovrd=off  block_type=logical
      settings: xl_area=[1 0 0 1 0 0 0]  block_version=VER_STRING_GOES_HERE
  Q : Outport
  wires:
  Delay/1 -> Inverter/1
  Inverter/1 -> Logical1/1
  Logical1/1 -> Q/1
  D/1 -> Delay/1, Logical1/2

== system wlan_phy_tx_pmd/Start Ctrl/Add TXEN Extension/S-R Latch1 ==
  S : Inport
  R : Inport  Port=2
  Constant1 : xbsIndex_r4/Constant  const=1  gui_display_data_type=Fixed-point  arith_type=Boolean  n_bits=1  bin_pt=0  preci_type=Single  exp_width=8  frac_width=24  explicit_period=off  period=1  equ=P=C  opselect=C  inp2=PCIN>>17  opr=+  inp1=P  carry=CIN  dbl_ovrd=off  block_type=constant
      settings: block_version=VER_STRING_GOES_HERE
  Convert1 : xbsIndex_r4/Convert  gui_display_data_type=Boolean  arith_type=Boolean  n_bits=1  bin_pt=0  float_type=Single  exp_bits=8  fraction_bits=24  quantization=Truncate  overflow=Wrap  en=off  latency=0  dbl_ovrd=off  pipeline=off  block_type=convert
  Convert2 : xbsIndex_r4/Convert  gui_display_data_type=Boolean  arith_type=Boolean  n_bits=1  bin_pt=0  float_type=Single  exp_bits=8  fraction_bits=24  quantization=Truncate  overflow=Wrap  en=off  latency=0  dbl_ovrd=off  pipeline=off  block_type=convert
  Register2 : xbsIndex_r4/Register  init=0  rst=on  en=on  dbl_ovrd=off  block_type=register
      settings: xl_area=[1 1 0 0 0 0 0]  block_version=VER_STRING_GOES_HERE
  Q : Outport
  wires:
  Convert2/1 -> Register2/3
  Convert1/1 -> Register2/2
  S/1 -> Convert2/1
  Register2/1 -> Q/1
  R/1 -> Convert1/1
  Constant1/1 -> Register2/1

== system wlan_phy_tx_pmd/Start Ctrl/Simulation Stop/Posedge3 ==
  note: Rising Edge Detection
  D : Inport
  Delay : xbsIndex_r4/Delay  rst=off  infoeditControl=Selection of Reset will increase slice count due to use of real FFs and instead of SRLs  en=off  latency=1  dbl_ovrd=off  reg_retiming=off  block_type=delay
      settings: infoedit=Hardware notes: A delay line is a chain, each link of which is an SRL16 followed by a flip-flop. If register retiming is enabled, the delay line is a chain of flip-flops.  xl_area=[1 1 0 0 0 0 0]  block_version=VER_STRING_GOES_HERE
  Inverter : xbsIndex_r4/Inverter  en=off  latency=0  dbl_ovrd=off  block_type=inv
      settings: xl_area=[0 0 0 0 0 0 0]  block_version=VER_STRING_GOES_HERE
  Logical1 : xbsIndex_r4/Logical  logical_function=AND  inputs=2  en=off  latency=0  precision=Full  arith_type=Unsigned  n_bits=8  bin_pt=2  align_bp=on  dbl_ovrd=off  block_type=logical
      settings: xl_area=[1 0 0 1 0 0 0]  block_version=VER_STRING_GOES_HERE
  Q : Outport
  wires:
  D/1 -> Logical1/2, Delay/1
  Logical1/1 -> Q/1
  Inverter/1 -> Logical1/1
  Delay/1 -> Inverter/1

== system wlan_phy_tx_pmd/Start Ctrl/Simulation Stop/S-R Latch1 ==
  S : Inport
  R : Inport  Port=2
  Constant1 : xbsIndex_r4/Constant  const=1  gui_display_data_type=Boolean  arith_type=Boolean  n_bits=1  bin_pt=0  preci_type=Single  exp_width=8  frac_width=24  explicit_period=off  period=1  equ=P=C  opselect=C  inp2=PCIN>>17  opr=+  inp1=P  carry=CIN  dbl_ovrd=off  block_type=constant
      settings: block_version=VER_STRING_GOES_HERE
  Convert1 : xbsIndex_r4/Convert  gui_display_data_type=Boolean  arith_type=Boolean  n_bits=1  bin_pt=0  float_type=Single  exp_bits=8  fraction_bits=24  quantization=Truncate  overflow=Wrap  en=off  latency=0  dbl_ovrd=off  pipeline=off  block_type=convert
  Convert2 : xbsIndex_r4/Convert  gui_display_data_type=Boolean  arith_type=Boolean  n_bits=1  bin_pt=0  float_type=Single  exp_bits=8  fraction_bits=24  quantization=Truncate  overflow=Wrap  en=off  latency=0  dbl_ovrd=off  pipeline=off  block_type=convert
  Register2 : xbsIndex_r4/Register  init=0  rst=on  en=on  dbl_ovrd=off  block_type=register
      settings: xl_area=[1 1 0 0 0 0 0]  block_version=VER_STRING_GOES_HERE
  Q : Outport
  wires:
  S/1 -> Convert2/1
  Register2/1 -> Q/1
  R/1 -> Convert1/1
  Constant1/1 -> Register2/1
  Convert1/1 -> Register2/2
  Convert2/1 -> Register2/3

== system wlan_phy_tx_pmd/Start Ctrl/Tx Active Debug Signal/Dly ==
  note: Need a delay of ~746 160MHz cycles
  note: Hold the signal High for 20 cycles
  note: This delay allows the Tx_Running debug output to directly trigger
      | pkt detection at another node. The delay value was measured in hardware
      | and corresponds to the latencies in the Tx/Rx circuits and the Rx processing
      | delay from first sample to pkt det firing.
  D : Inport
  Constant : xbsIndex_r4/Constant  const=745  gui_display_data_type=Fixed-point  arith_type=Unsigned  n_bits=16  bin_pt=0  preci_type=Single  exp_width=8  frac_width=24  explicit_period=off  period=1  equ=P=C  opselect=C  inp2=PCIN>>17  opr=+  inp1=P  carry=CIN  dbl_ovrd=off  block_type=constant
  Constant1 : xbsIndex_r4/Constant  const=20  gui_display_data_type=Fixed-point  arith_type=Unsigned  n_bits=8  bin_pt=0  preci_type=Single  exp_width=8  frac_width=24  explicit_period=off  period=1  equ=P=C  opselect=C  inp2=PCIN>>17  opr=+  inp1=P  carry=CIN  dbl_ovrd=off  block_type=constant
  Convert : xbsIndex_r4/Convert  gui_display_data_type=Boolean  arith_type=Boolean  n_bits=16  bin_pt=14  float_type=Single  exp_bits=8  fraction_bits=24  quantization=Truncate  overflow=Wrap  en=off  latency=0  dbl_ovrd=off  pipeline=off  block_type=convert
  Convert1 : xbsIndex_r4/Convert  gui_display_data_type=Boolean  arith_type=Boolean  n_bits=16  bin_pt=14  float_type=Single  exp_bits=8  fraction_bits=24  quantization=Truncate  overflow=Wrap  en=off  latency=0  dbl_ovrd=off  pipeline=off  block_type=convert
  Convert2 : xbsIndex_r4/Convert  gui_display_data_type=Fixed-point  arith_type=Unsigned  n_bits=1  bin_pt=0  float_type=Single  exp_bits=8  fraction_bits=24  quantization=Truncate  overflow=Wrap  en=off  latency=0  dbl_ovrd=off  pipeline=off  block_type=convert
  Counter : xbsIndex_r4/Counter  cnt_type=Free Running  cnt_to=Inf  operation=Up  start_count=0  cnt_by_val=1  arith_type=Unsigned  n_bits=10  bin_pt=0  load_pin=off  rst=on  en=on  explicit_period=off  period=1  dbl_ovrd=off  use_behavioral_HDL=off  implementation=Fabric  block_type=counter
  Counter1 : xbsIndex_r4/Counter  cnt_type=Free Running  cnt_to=Inf  operation=Up  start_count=0  cnt_by_val=1  arith_type=Unsigned  n_bits=5  bin_pt=0  load_pin=off  rst=on  en=on  explicit_period=on  period=1  dbl_ovrd=off  use_behavioral_HDL=off  implementation=Fabric  block_type=counter
  Relational : xbsIndex_r4/Relational  mode=a>=b  en=off  latency=0  dbl_ovrd=off  block_type=relational
  Relational1 : xbsIndex_r4/Relational  mode=a>=b  en=off  latency=0  dbl_ovrd=off  block_type=relational
  S-R Latch1 : Subsystem
  S-R Latch2 : Subsystem
  Q : Outport
  wires:
  D/1 -> S-R Latch2/1(S)
  S-R Latch2/1(Q) -> Convert1/1
  Constant/1 -> Relational/2
  Counter/1 -> Relational/1
  S-R Latch1/1(Q) -> Convert/1, Convert2/1
  Relational1/1 -> Counter/1, S-R Latch2/2(R), S-R Latch1/2(R), Counter1/1
  Constant1/1 -> Relational1/2
  Counter1/1 -> Relational1/1
  Relational/1 -> S-R Latch1/1(S)
  Convert/1 -> Counter1/2
  Convert1/1 -> Counter/2
  Convert2/1 -> Q/1

== system wlan_phy_tx_pmd/IFFT and Cyclic Prefix/Buffer and Cyclic Prefix/Control/S-R Latch1 ==
  S : Inport
  R : Inport  Port=2
  Constant1 : xbsIndex_r4/Constant  const=1  gui_display_data_type=Fixed-point  arith_type=Boolean  n_bits=1  bin_pt=0  preci_type=Single  exp_width=8  frac_width=24  explicit_period=off  period=1  equ=P=C  opselect=C  inp2=PCIN>>17  opr=+  inp1=P  carry=CIN  dbl_ovrd=off  block_type=constant
      settings: block_version=VER_STRING_GOES_HERE
  Convert1 : xbsIndex_r4/Convert  gui_display_data_type=Boolean  arith_type=Boolean  n_bits=1  bin_pt=0  float_type=Single  exp_bits=8  fraction_bits=24  quantization=Truncate  overflow=Wrap  en=off  latency=0  dbl_ovrd=off  pipeline=off  block_type=convert
  Convert2 : xbsIndex_r4/Convert  gui_display_data_type=Boolean  arith_type=Boolean  n_bits=1  bin_pt=0  float_type=Single  exp_bits=8  fraction_bits=24  quantization=Truncate  overflow=Wrap  en=off  latency=0  dbl_ovrd=off  pipeline=off  block_type=convert
  Register2 : xbsIndex_r4/Register  init=0  rst=on  en=on  dbl_ovrd=off  block_type=register
      settings: xl_area=[1 1 0 0 0 0 0]  block_version=VER_STRING_GOES_HERE
  Q : Outport
  wires:
  S/1 -> Convert2/1
  Register2/1 -> Q/1
  R/1 -> Convert1/1
  Constant1/1 -> Register2/1
  Convert1/1 -> Register2/2
  Convert2/1 -> Register2/3

== system wlan_phy_tx_pmd/PSDU Syms Gen/Index Gen/Bits Per Sym/S-R Latch1 ==
  S : Inport
  R : Inport  Port=2
  Constant1 : xbsIndex_r4/Constant  const=1  gui_display_data_type=Fixed-point  arith_type=Boolean  n_bits=1  bin_pt=0  preci_type=Single  exp_width=8  frac_width=24  explicit_period=off  period=1  equ=P=C  opselect=C  inp2=PCIN>>17  opr=+  inp1=P  carry=CIN  dbl_ovrd=off  block_type=constant
      settings: block_version=VER_STRING_GOES_HERE
  Convert1 : xbsIndex_r4/Convert  gui_display_data_type=Boolean  arith_type=Boolean  n_bits=1  bin_pt=0  float_type=Single  exp_bits=8  fraction_bits=24  quantization=Truncate  overflow=Wrap  en=off  latency=0  dbl_ovrd=off  pipeline=off  block_type=convert
  Convert2 : xbsIndex_r4/Convert  gui_display_data_type=Boolean  arith_type=Boolean  n_bits=1  bin_pt=0  float_type=Single  exp_bits=8  fraction_bits=24  quantization=Truncate  overflow=Wrap  en=off  latency=0  dbl_ovrd=off  pipeline=off  block_type=convert
  Register2 : xbsIndex_r4/Register  init=0  rst=on  en=on  dbl_ovrd=off  block_type=register
      settings: xl_area=[1 1 0 0 0 0 0]  block_version=VER_STRING_GOES_HERE
  Q : Outport
  wires:
  Convert2/1 -> Register2/3
  Convert1/1 -> Register2/2
  Constant1/1 -> Register2/1
  R/1 -> Convert1/1
  Register2/1 -> Q/1
  S/1 -> Convert2/1
